simulink model "part_A_q12"  (R2023b)
settings: Solver=VariableStepAuto  StartTime=0.0  StopTime=15  RelTol=1e-3
values from neighbouring files (symbols this model uses):
  A = [   zeros(7)    eye(7) ... (first row only)    [FOUND_full_car.m]    (also in part_A_q12_init.m = [0, 1; -k/m, -c/m]; q14_15.m = [0, 1, 0, -1;      -ks/ms, -bs/ms, 0, bs/ms;      0, 0, 0, 1; q5.m = [0, 1; -k/m, -c/m]; q7.m = [0, 1; -k/m, -c/m])
  B = [   zeros(7,4) ... (first row only)    [FOUND_full_car.m]    (also in part_A_q12_init.m = [0; 1/m]; q14_15.m = [0;      1/ms;      0;      -1/mu]; q5.m = [0; 1/m]; q7.m = [0; 1/m])
  c = 1000    [init_params.m]
  K = [   k11     k12     k13     -kf     -kf     -kr     -kr ... (first row only)    [FOUND_full_car.m]
  k = 16000    [init_params.m]
  L = [-1; c/m]    [part_A_q12_init.m]    (also in part_C_q17.m = [0;      0;      -1;      0]; q14_15.m = [0;      0;      -1;      0]; q5.m; q7.m)
  m = 840    [FOUND_full_car.m]    (also in init_params.m = 240)
settings Model: Creator=yusufcagriogut  LastModifiedBy=yusufcagriogut

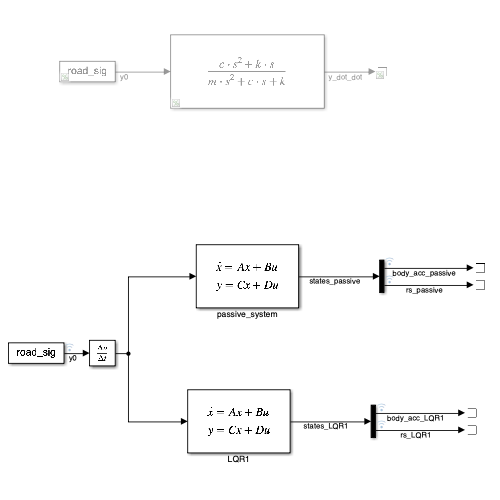
[thumbnail: Simulink's stored preview of the top-level diagram]
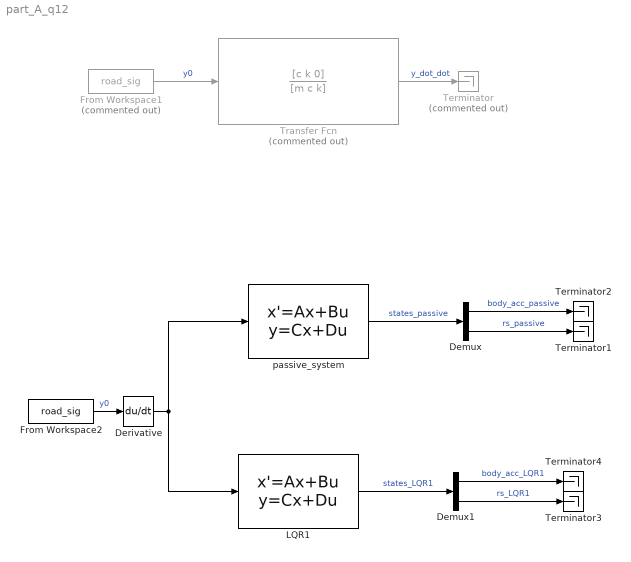
== system part_A_q12 ==
  Demux : Demux  Outputs=2
  Demux1 : Demux  Outputs=2
  Derivative : Derivative
  From Workspace1 : FromWorkspace  Commented=on  VariableName=road_sig
  From Workspace2 : FromWorkspace  VariableName=road_sig
  LQR1 : StateSpace  A=A-B*K  B=L  C=A  D=[0;0]  InitialCondition=0
  Terminator : Terminator  Commented=on
  Terminator{1..4} (4 alike) : Terminator
  Transfer Fcn : TransferFcn  Commented=on  Numerator=[c k 0]  Denominator=[m c k]
  passive_system : StateSpace  A=A  B=L  C=A  D=[0;0]  InitialCondition=0
  wires:
  From Workspace1/1 -> Transfer Fcn/1  "y0"
  Transfer Fcn/1 -> Terminator/1  "y_dot_dot"
  From Workspace2/1 -> Derivative/1  "y0"
  passive_system/1 -> Demux/1  "states_passive"
  Demux/1 -> Terminator2/1  "body_acc_passive"
  Demux/2 -> Terminator1/1  "rs_passive"
  LQR1/1 -> Demux1/1  "states_LQR1"
  Demux1/2 -> Terminator3/1  "rs_LQR1"
  Demux1/1 -> Terminator4/1  "body_acc_LQR1"
  Derivative/1 -> passive_system/1, LQR1/1
